simulink model "Fig58"  (R2014b)
settings: Solver=ode3  StartTime=0.0  StopTime=.064  FixedStep=1e-3  RelTol=1e-3
libraries: commseqgen2 x1, simulink_extras x1
settings Model: Creator=Silage  LastModifiedBy=Silage

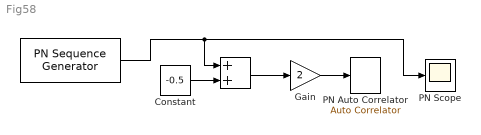
== system Fig58 ==
  " " : commseqgen2/PN Sequence Generator  poly=[1 0 0 1 1]  ini_sta=[1 0 0 1]  outBitMaskSource=Dialog parameter  shift=0  outVarSiz=off  maxOutSizeMode=Dialog parameter  maxOutSize=[10 1]  Ts=1e-3  frameBased=off  sampPerFrame=1  reset=off  bitPackedOutputs=off  outDataType=double  numPackedBits=8  bitPackDataSigned=off  bitPackedOutDType=double
  "    " : Sum
  " PN Scope" : Scope
      settings: YMin=-0.5  YMax=1.5
  Constant : Constant  Value=-0.5
  Gain : Gain  Gain=2
  PN Auto Correlator : simulink_extras/Additional Sinks/Auto Correlator  npts=64  HowOften=64  sampleT=1e-3
  wires:
  " "/1 -> " PN Scope"/1, "    "/1
  Constant/1 -> "    "/2
  "    "/1 -> Gain/1
  Gain/1 -> PN Auto Correlator/1
